simulink model "tqdtqr_rebuild_V3"  (R2021b)
settings: Solver=VariableStepAuto  StartTime=0.0  StopTime=10.0  RelTol=1e-3
undefined symbols (not defined in the file): ATQD_AfterTqMinGain_X_Deg, ATQD_APSCreepBaseTqD_X_kph, ATQD_APSCreepBaseTqD_Y_Deg, ATQD_APSCreepBaseTqR_X_kph, ATQD_APSCreepBaseTqR_Y_Deg, ATQD_APSCreepIterm_X_kph, ATQD_APSCreepIterm_Y_kph, ATQD_APSCreepPterm_X_kph, ATQD_APSCreepPterm_Y_kph, ATQD_APSDecReq_X_kph, ATQD_APSDecReq_Y_mps2, ATQD_APSDecReqCMD_X_kph, ATQD_APSDecReqTs_X_pct, ATQD_APSDecTimeGain_X_Deg, ATQD_APSDecTimeGain_Y_s, ATQD_APSReqLowSpd_X_Deg, ATQD_AutoHoldReleaseBPS_X_Deg, ATQD_AWDLoadTrqnsGain_X_kg, ATQD_AWDLoadTrqnsGain_Y_pct, ATQD_BOSEnBPSPosn_X_kph, ATQD_BOSMap_X_rpm, ATQD_BOSMap_Y_pct, ATQD_CreepBaseTqD_X_kph, ATQD_CreepBaseTqD_Y_Deg, ATQD_CreepBaseTqR_X_kph, ATQD_CreepBaseTqR_Y_Deg, ATQD_CreepBPSDisPosn_X_Deg, ATQD_CreepBPSDisPosnR_X_Deg, ATQD_CreepBPSEnPosn_X_Deg, ATQD_CreepBPSEnPosnR_X_Deg, ATQD_CreepDeltaTq_X_kph, ATQD_CreepIterm_X_kph, ATQD_CreepIterm_Y_kph, ATQD_CreepItermMaxLimit_X_pct, ATQD_CreepPreloadTime_X_kph, ATQD_CreepPreloadTq_X_kph, ATQD_CreepPreloadTq_Y_s, ATQD_CreepProtTq_X_Deg, ATQD_CreepPterm_X_kph, ATQD_CreepPterm_Y_kph, ATQD_CreepRrTqSpRat_X_rpm, ATQD_CreepRrTqSpRat_Y_Nm, ATQD_CreepTargetSpdD_X_pct, ATQD_CreepTargetSpdR_X_pct, ATQD_CreepUpLimitTq_X_rpm, ATQD_DecIneOPDHoldEnDelay_X_Deg, ATQD_DecIneOPDHoldEnDelay_Y_bar, ATQD_ECOTqMapD_X_rpm, ATQD_ECOTqMapD_Y_pct, ATQD_EMTqMapD_X_rpm, ATQD_EMTqMapD_Y_pct, ATQD_EOPDTqMapDCon_X_rpm, ATQD_EOPDTqMapDCon_Y_Deg, ATQD_EstInitVehWeight_X_c, ATQD_FAfterTqCMDGain_X_rpm, ATQD_FAfterTqCMDGain_Y_pct, ATQD_ForceLowSpd_X_Deg, ATQD_ForcePLimitSpd_X_Deg, ATQD_FrLossMAPLowV_X_rpm, ATQD_FrLossMAPLowV_Y_Nm ... (+949)
libraries: simulink x235, hcu_lib x208, tqr x63, tqd x6
(part 26 of 37)

== system tqdtqr_rebuild_V3/Input_Convert/Main function/DriverWhlTqDem function/Driver mode determination/NOLHM ShiftD NRM LV5 ==
  VTQD_ActAPSPosn_pct : Inport
  VTQD_TqTargetShaftSpd_rpm : Inport  Port=2
  VTQD_RL5TqMapDComp_Nm : Inport  Port=3
  Enable : EnablePort
  Add : Sum
  MTQD_NL5TqMapD_Z_Nm1 : Lookup_n-D  BreakpointsForDimension1=ATQD_NL1TqMapD_Y_pct  BreakpointsForDimension2=ATQD_NL1TqMapD_X_rpm  Table=MTQD_NL5TqMapD_Z_Nm  ExtrapMethod=Clip  InternalRulePriority=Speed  RndMeth=Simplest  InputSameDT=on
      settings: InputPortMap=u0,u1
  VTQD_NL5TqMapDOut_Nm : Outport
  wires:
  MTQD_NL5TqMapD_Z_Nm1/1 -> [VTQD_NL5TqMapD_Nm]
  [VTQD_TqTargetShaftSpd_rpm] -> MTQD_NL5TqMapD_Z_Nm1/2
  [VTQD_ActAPSPosn_pct] -> MTQD_NL5TqMapD_Z_Nm1/1
  VTQD_ActAPSPosn_pct/1 -> [VTQD_ActAPSPosn_pct]
  VTQD_TqTargetShaftSpd_rpm/1 -> [VTQD_TqTargetShaftSpd_rpm]
  [VTQD_NL5TqMapD_Nm] -> Add/2
  [VTQD_RL5TqMapDComp_Nm] -> Add/1
  Add/1 -> VTQD_NL5TqMapDOut_Nm/1
  VTQD_RL5TqMapDComp_Nm/1 -> [VTQD_RL5TqMapDComp_Nm]

== system tqdtqr_rebuild_V3/Input_Convert/Main function/DriverWhlTqDem function/Driver mode determination/NOLHM ShiftD NRM OPD ==
  VTQD_ActAPSPosn_pct : Inport
  VTQD_TqTargetShaftSpd_rpm : Inport  Port=2
  VVMC_EstSlope_Deg : Inport  Port=3
  VTQD_APSReqTimer_s : Inport  Port=4
  VTQD_LowIdleAccPedal_flg : Inport  Port=5
  VTQD_OPDHoldEnRel_flg : Inport  Port=6
  VTQD_OPDHoldActRelTq_Nm : Inport  Port=7
  VTQD_VehActSpd_kph : Inport  Port=8
  VTQD_SlopeUp_flg : Inport  Port=9
  Enable : EnablePort
  AND : Logic  AllPortsSameDT=off  OutDataTypeStr=boolean
  Add : Sum
  Constant1 : Constant  Value=ZERO_FLOAT
  Constant2 : Constant  Value=KTQD_OPDHTqDisComSpd_kph
  Constant3 : Constant  Value=KTQD_OPDHTqDisAPSPosn_pct
  Constant9 : Constant  Value=KTQD_APSReqDelayTime_s
  Detect Increase : simulink/Logic and Bit Operations/Detect Increase  vinit=0.0  OutDataTypeStr=boolean
  MTQD_NOPDTqMapDCon_Z_Nm : Lookup_n-D  BreakpointsForDimension1=ATQD_NOPDTqMapDCon_Y_Deg  BreakpointsForDimension2=ATQD_NOPDTqMapDCon_X_rpm  Table=MTQD_NOPDTqMapDCon_Z_Nm  ExtrapMethod=Clip  InternalRulePriority=Speed  RndMeth=Simplest  InputSameDT=on
      settings: InputPortMap=u0,u1
  MTQD_NOPDTqMapD_Z_Nm1 : Lookup_n-D  BreakpointsForDimension1=ATQD_NL1TqMapD_Y_pct  BreakpointsForDimension2=ATQD_NL1TqMapD_X_rpm  Table=MTQD_NOPDTqMapD_Z_Nm  ExtrapMethod=Clip  InternalRulePriority=Speed  RndMeth=Simplest  InputSameDT=on
      settings: InputPortMap=u0,u1
  Max : MinMax  Function=max  Inputs=2
  NOT : Logic  Operator=NOT  AllPortsSameDT=off  OutDataTypeStr=boolean
  OR : Logic  Operator=OR  Inputs=3  AllPortsSameDT=off  OutDataTypeStr=boolean
  OR1 : Logic  Operator=OR  AllPortsSameDT=off  OutDataTypeStr=boolean
  Relational Operator : RelationalOperator  Operator=>  OutDataTypeStr=boolean  RndMeth=Simplest
  Relational Operator1 : RelationalOperator  OutDataTypeStr=boolean  RndMeth=Simplest
  Relational Operator2 : RelationalOperator  OutDataTypeStr=boolean  RndMeth=Simplest
  SR_Latch : hcu_lib/Basic_Blocks/SR_Latch
  Switch : Switch  Criteria=u2 ~= 0
      settings: AttributesFormatString=%<Criteria>
  Switch1 : Switch  Criteria=u2 ~= 0
      settings: AttributesFormatString=%<Criteria>
  VTQD_NOPDTqMapDOut_Nm : Outport
  wires:
  MTQD_NOPDTqMapD_Z_Nm1/1 -> [VTQD_NOPDTqMapD_Nm]
  [VTQD_ActAPSPosn_pct] -> MTQD_NOPDTqMapD_Z_Nm1/1
  [VTQD_TqTargetShaftSpd_rpm] -> MTQD_NOPDTqMapD_Z_Nm1/2
  [VVMC_EstSlope_Deg] -> MTQD_NOPDTqMapDCon_Z_Nm/1
  [VTQD_TqTargetShaftSpd_rpm] -> MTQD_NOPDTqMapDCon_Z_Nm/2
  MTQD_NOPDTqMapDCon_Z_Nm/1 -> [VTQD_NOPDTqMapDCon_Nm]
  VTQD_ActAPSPosn_pct/1 -> [VTQD_ActAPSPosn_pct]
  VTQD_TqTargetShaftSpd_rpm/1 -> [VTQD_TqTargetShaftSpd_rpm]
  VVMC_EstSlope_Deg/1 -> [VVMC_EstSlope_Deg]
  VTQD_APSReqTimer_s/1 -> [VTQD_APSReqTimer_s]
  VTQD_LowIdleAccPedal_flg/1 -> [VTQD_LowIdleAccPedal_flg]
  VTQD_OPDHoldEnRel_flg/1 -> [VTQD_OPDHoldEnRel_flg]
  VTQD_OPDHoldActRelTq_Nm/1 -> [VTQD_OPDHoldActRelTq_Nm]
  VTQD_VehActSpd_kph/1 -> [VTQD_VehActSpd_kph]
  VTQD_SlopeUp_flg/1 -> [VTQD_SlopeUp_flg]
  AND/1 -> OR1/1
  Constant3/1 -> Relational Operator1/2
  [VTQD_ActAPSPosn_pct] -> Relational Operator1/1
  Constant1/1 -> Switch/1
  [VTQD_LowIdleAccPedal_flg] -> OR/1
  OR1/1 -> Switch/2
  NOT/1 -> OR/3
  Max/1 -> Switch1/1
  [VTQD_LowIdleAccPedal_flg] -> AND/2
  Relational Operator/1 -> OR/2
  Constant2/1 -> Relational Operator/2
  Relational Operator2/1 -> AND/1
  [VTQD_NOPDTqMapD_Nm] -> Add/1
  [VTQD_APSReqTimer_s] -> Relational Operator2/1
  OR/1 -> SR_Latch/2
  Relational Operator1/1 -> OR1/2
  Detect Increase/1 -> SR_Latch/1
  Constant9/1 -> Relational Operator2/2
  Add/1 -> Max/1, Switch1/3  "VTQD_NOPDActTqMapD_Nm"
  SR_Latch/1 -> Switch1/2  "VTQD_OPDHoldRelPedTq_flg"
  Switch/1 -> Add/2
  [VTQD_NOPDTqMapDCon_Nm] -> Switch/3
  [VTQD_OPDHoldActRelTq_Nm] -> Max/2
  [VTQD_OPDHoldEnRel_flg] -> Detect Increase/1
  [VTQD_VehActSpd_kph] -> Relational Operator/1
  [VTQD_SlopeUp_flg] -> NOT/1
  Switch1/1 -> VTQD_NOPDTqMapDOut_Nm/1

== system tqdtqr_rebuild_V3/Input_Convert/Main function/DriverWhlTqDem function/Driver mode determination/NOLHM ShiftD Sport Invalid ==
  VTQD_ActAPSPosn_pct : Inport
  VTQD_TqTargetShaftSpd_rpm : Inport  Port=2
  Enable : EnablePort
  MTQD_SL1TqMapD_Z_Nm : Lookup_n-D  BreakpointsForDimension1=ATQD_SL1TqMapD_Y_pct  BreakpointsForDimension2=ATQD_SL1TqMapD_X_rpm  Table=MTQD_SL1TqMapD_Z_Nm  ExtrapMethod=Clip  InternalRulePriority=Speed  RndMeth=Simplest  InputSameDT=on
      settings: InputPortMap=u0,u1
  VTQD_SLTqMapDOutInv_Nm : Outport
  wires:
  MTQD_SL1TqMapD_Z_Nm/1 -> [VTQD_SL1TqMapD_Nm]
  [VTQD_TqTargetShaftSpd_rpm] -> MTQD_SL1TqMapD_Z_Nm/2
  [VTQD_ActAPSPosn_pct] -> MTQD_SL1TqMapD_Z_Nm/1
  VTQD_ActAPSPosn_pct/1 -> [VTQD_ActAPSPosn_pct]
  VTQD_TqTargetShaftSpd_rpm/1 -> [VTQD_TqTargetShaftSpd_rpm]
  [VTQD_SL1TqMapD_Nm] -> VTQD_SLTqMapDOutInv_Nm/1

== system tqdtqr_rebuild_V3/Input_Convert/Main function/DriverWhlTqDem function/Driver mode determination/NOLHM ShiftD Sport LV1 ==
  VTQD_ActAPSPosn_pct : Inport
  VTQD_TqTargetShaftSpd_rpm : Inport  Port=2
  VTQD_RL1TqMapDComp_Nm : Inport  Port=3
  Enable : EnablePort
  Add : Sum
  MTQD_SL1TqMapD_Z_Nm : Lookup_n-D  BreakpointsForDimension1=ATQD_SL1TqMapD_Y_pct  BreakpointsForDimension2=ATQD_SL1TqMapD_X_rpm  Table=MTQD_SL1TqMapD_Z_Nm  ExtrapMethod=Clip  InternalRulePriority=Speed  RndMeth=Simplest  InputSameDT=on
      settings: InputPortMap=u0,u1
  VTQD_SL1TqMapDOut_Nm : Outport
  wires:
  MTQD_SL1TqMapD_Z_Nm/1 -> [VTQD_SL1TqMapD_Nm]
  [VTQD_TqTargetShaftSpd_rpm] -> MTQD_SL1TqMapD_Z_Nm/2
  [VTQD_ActAPSPosn_pct] -> MTQD_SL1TqMapD_Z_Nm/1
  [VTQD_SL1TqMapD_Nm] -> Add/2
  [VTQD_RL1TqMapDComp_Nm] -> Add/1
  Add/1 -> VTQD_SL1TqMapDOut_Nm/1
  VTQD_ActAPSPosn_pct/1 -> [VTQD_ActAPSPosn_pct]
  VTQD_TqTargetShaftSpd_rpm/1 -> [VTQD_TqTargetShaftSpd_rpm]
  VTQD_RL1TqMapDComp_Nm/1 -> [VTQD_RL1TqMapDComp_Nm]

== system tqdtqr_rebuild_V3/Input_Convert/Main function/DriverWhlTqDem function/Driver mode determination/NOLHM ShiftD Sport LV2 ==
  VTQD_ActAPSPosn_pct : Inport
  VTQD_TqTargetShaftSpd_rpm : Inport  Port=2
  VTQD_RL2TqMapDComp_Nm : Inport  Port=3
  Enable : EnablePort
  Add : Sum
  MTQD_SL2TqMapD_Z_Nm : Lookup_n-D  BreakpointsForDimension1=ATQD_SL1TqMapD_Y_pct  BreakpointsForDimension2=ATQD_SL1TqMapD_X_rpm  Table=MTQD_SL2TqMapD_Z_Nm  ExtrapMethod=Clip  InternalRulePriority=Speed  RndMeth=Simplest  InputSameDT=on
      settings: InputPortMap=u0,u1
  VTQD_SL2TqMapDOut_Nm : Outport
  wires:
  [VTQD_ActAPSPosn_pct] -> MTQD_SL2TqMapD_Z_Nm/1
  MTQD_SL2TqMapD_Z_Nm/1 -> [VTQD_SL2TqMapD_Nm]
  [VTQD_TqTargetShaftSpd_rpm] -> MTQD_SL2TqMapD_Z_Nm/2
  VTQD_ActAPSPosn_pct/1 -> [VTQD_ActAPSPosn_pct]
  VTQD_TqTargetShaftSpd_rpm/1 -> [VTQD_TqTargetShaftSpd_rpm]
  [VTQD_RL2TqMapDComp_Nm] -> Add/1
  [VTQD_SL2TqMapD_Nm] -> Add/2
  Add/1 -> VTQD_SL2TqMapDOut_Nm/1
  VTQD_RL2TqMapDComp_Nm/1 -> [VTQD_RL2TqMapDComp_Nm]

== system tqdtqr_rebuild_V3/Input_Convert/Main function/DriverWhlTqDem function/Driver mode determination/NOLHM ShiftD Sport LV3 ==
  VTQD_ActAPSPosn_pct : Inport
  VTQD_TqTargetShaftSpd_rpm : Inport  Port=2
  VTQD_RL3TqMapDComp_Nm : Inport  Port=3
  Enable : EnablePort
  Add : Sum
  MTQD_SL3TqMapD_Z_Nm : Lookup_n-D  BreakpointsForDimension1=ATQD_SL1TqMapD_Y_pct  BreakpointsForDimension2=ATQD_SL1TqMapD_X_rpm  Table=MTQD_SL3TqMapD_Z_Nm  ExtrapMethod=Clip  InternalRulePriority=Speed  RndMeth=Simplest  InputSameDT=on
      settings: InputPortMap=u0,u1
  VTQD_SL3TqMapDOut_Nm : Outport
  wires:
  [VTQD_TqTargetShaftSpd_rpm] -> MTQD_SL3TqMapD_Z_Nm/2
  [VTQD_ActAPSPosn_pct] -> MTQD_SL3TqMapD_Z_Nm/1
  MTQD_SL3TqMapD_Z_Nm/1 -> [VTQD_SL3TqMapD_Nm]
  VTQD_ActAPSPosn_pct/1 -> [VTQD_ActAPSPosn_pct]
  VTQD_TqTargetShaftSpd_rpm/1 -> [VTQD_TqTargetShaftSpd_rpm]
  Add/1 -> VTQD_SL3TqMapDOut_Nm/1
  [VTQD_RL3TqMapDComp_Nm] -> Add/1
  [VTQD_SL3TqMapD_Nm] -> Add/2
  VTQD_RL3TqMapDComp_Nm/1 -> [VTQD_RL3TqMapDComp_Nm]

== system tqdtqr_rebuild_V3/Input_Convert/Main function/DriverWhlTqDem function/Driver mode determination/NOLHM ShiftD Sport LV4 ==
  VTQD_ActAPSPosn_pct : Inport
  VTQD_TqTargetShaftSpd_rpm : Inport  Port=2
  VTQD_RL4TqMapDComp_Nm : Inport  Port=3
  Enable : EnablePort
  Add : Sum
  MTQD_SL4TqMapD_Z_Nm : Lookup_n-D  BreakpointsForDimension1=ATQD_SL1TqMapD_Y_pct  BreakpointsForDimension2=ATQD_SL1TqMapD_X_rpm  Table=MTQD_SL4TqMapD_Z_Nm  ExtrapMethod=Clip  InternalRulePriority=Speed  RndMeth=Simplest  InputSameDT=on
      settings: InputPortMap=u0,u1
  VTQD_SL4TqMapDOut_Nm : Outport
  wires:
  [VTQD_ActAPSPosn_pct] -> MTQD_SL4TqMapD_Z_Nm/1
  MTQD_SL4TqMapD_Z_Nm/1 -> [VTQD_SL4TqMapD_Nm]
  [VTQD_TqTargetShaftSpd_rpm] -> MTQD_SL4TqMapD_Z_Nm/2
  VTQD_ActAPSPosn_pct/1 -> [VTQD_ActAPSPosn_pct]
  VTQD_TqTargetShaftSpd_rpm/1 -> [VTQD_TqTargetShaftSpd_rpm]
  [VTQD_RL4TqMapDComp_Nm] -> Add/1
  [VTQD_SL4TqMapD_Nm] -> Add/2
  Add/1 -> VTQD_SL4TqMapDOut_Nm/1
  VTQD_RL4TqMapDComp_Nm/1 -> [VTQD_RL4TqMapDComp_Nm]

== system tqdtqr_rebuild_V3/Input_Convert/Main function/DriverWhlTqDem function/Driver mode determination/NOLHM ShiftD Sport LV5 ==
  VTQD_ActAPSPosn_pct : Inport
  VTQD_TqTargetShaftSpd_rpm : Inport  Port=2
  VTQD_RL5TqMapDComp_Nm : Inport  Port=3
  Enable : EnablePort
  Add : Sum
  MTQD_SL5TqMapD_Z_Nm : Lookup_n-D  BreakpointsForDimension1=ATQD_SL1TqMapD_Y_pct  BreakpointsForDimension2=ATQD_SL1TqMapD_X_rpm  Table=MTQD_SL5TqMapD_Z_Nm  ExtrapMethod=Clip  InternalRulePriority=Speed  RndMeth=Simplest  InputSameDT=on
      settings: InputPortMap=u0,u1
  VTQD_SL5TqMapDOut_Nm : Outport
  wires:
  MTQD_SL5TqMapD_Z_Nm/1 -> [VTQD_SL5TqMapD_Nm]
  [VTQD_TqTargetShaftSpd_rpm] -> MTQD_SL5TqMapD_Z_Nm/2
  [VTQD_ActAPSPosn_pct] -> MTQD_SL5TqMapD_Z_Nm/1
  VTQD_ActAPSPosn_pct/1 -> [VTQD_ActAPSPosn_pct]
  VTQD_TqTargetShaftSpd_rpm/1 -> [VTQD_TqTargetShaftSpd_rpm]
  [VTQD_RL5TqMapDComp_Nm] -> Add/1
  [VTQD_SL5TqMapD_Nm] -> Add/2
  Add/1 -> VTQD_SL5TqMapDOut_Nm/1
  VTQD_RL5TqMapDComp_Nm/1 -> [VTQD_RL5TqMapDComp_Nm]

== system tqdtqr_rebuild_V3/Input_Convert/Main function/DriverWhlTqDem function/Driver mode determination/NOLHM ShiftD Sport OPD ==
  VTQD_ActAPSPosn_pct : Inport
  VTQD_TqTargetShaftSpd_rpm : Inport  Port=2
  VVMC_EstSlope_Deg : Inport  Port=3
  VTQD_APSReqTimer_s : Inport  Port=4
  VTQD_LowIdleAccPedal_flg : Inport  Port=5
  VTQD_OPDHoldEnRel_flg : Inport  Port=6
  VTQD_OPDHoldActRelTq_Nm : Inport  Port=7
  VTQD_VehActSpd_kph : Inport  Port=8
  VTQD_SlopeUp_flg : Inport  Port=9
  Enable : EnablePort
  AND : Logic  AllPortsSameDT=off  OutDataTypeStr=boolean
  Add : Sum
  Constant1 : Constant  Value=ZERO_FLOAT
  Constant2 : Constant  Value=KTQD_OPDHTqDisComSpd_kph
  Constant4 : Constant  Value=KTQD_OPDHTqDisAPSPosn_pct
  Constant9 : Constant  Value=KTQD_APSReqDelayTime_s
  Detect Increase : simulink/Logic and Bit Operations/Detect Increase  vinit=0.0  OutDataTypeStr=boolean
  MTQD_SOPDTqMapDCon_Z_Nm : Lookup_n-D  BreakpointsForDimension1=ATQD_SOPDTqMapDCon_Y_Deg  BreakpointsForDimension2=ATQD_SOPDTqMapDCon_X_rpm  Table=MTQD_SOPDTqMapDCon_Z_Nm  ExtrapMethod=Clip  InternalRulePriority=Speed  RndMeth=Simplest  InputSameDT=on
      settings: InputPortMap=u0,u1
  MTQD_SOPDTqMapD_Z_Nm : Lookup_n-D  BreakpointsForDimension1=ATQD_SL1TqMapD_Y_pct  BreakpointsForDimension2=ATQD_SL1TqMapD_X_rpm  Table=MTQD_SOPDTqMapD_Z_Nm  ExtrapMethod=Clip  InternalRulePriority=Speed  RndMeth=Simplest  InputSameDT=on
      settings: InputPortMap=u0,u1
  Max : MinMax  Function=max  Inputs=2
  NOT : Logic  Operator=NOT  AllPortsSameDT=off  OutDataTypeStr=boolean
  OR : Logic  Operator=OR  Inputs=3  AllPortsSameDT=off  OutDataTypeStr=boolean
  OR1 : Logic  Operator=OR  AllPortsSameDT=off  OutDataTypeStr=boolean
  Relational Operator : RelationalOperator  Operator=>  OutDataTypeStr=boolean  RndMeth=Simplest
  Relational Operator2 : RelationalOperator  OutDataTypeStr=boolean  RndMeth=Simplest
  Relational Operator3 : RelationalOperator  OutDataTypeStr=boolean  RndMeth=Simplest
  SR_Latch : hcu_lib/Basic_Blocks/SR_Latch
  Switch : Switch  Criteria=u2 ~= 0
      settings: AttributesFormatString=%<Criteria>
  Switch1 : Switch  Criteria=u2 ~= 0
      settings: AttributesFormatString=%<Criteria>
  VTQD_SOPDTqMapDOut_Nm : Outport
  wires:
  MTQD_SOPDTqMapD_Z_Nm/1 -> [VTQD_SOPDTqMapD_Nm]
  [VVMC_EstSlope_Deg] -> MTQD_SOPDTqMapDCon_Z_Nm/1
  [VTQD_TqTargetShaftSpd_rpm] -> MTQD_SOPDTqMapDCon_Z_Nm/2
  MTQD_SOPDTqMapDCon_Z_Nm/1 -> [VTQD_SOPDTqMapDCon_Nm]
  [VTQD_ActAPSPosn_pct] -> MTQD_SOPDTqMapD_Z_Nm/1
  [VTQD_TqTargetShaftSpd_rpm] -> MTQD_SOPDTqMapD_Z_Nm/2
  VTQD_ActAPSPosn_pct/1 -> [VTQD_ActAPSPosn_pct]
  VTQD_TqTargetShaftSpd_rpm/1 -> [VTQD_TqTargetShaftSpd_rpm]
  VVMC_EstSlope_Deg/1 -> [VVMC_EstSlope_Deg]
  [VTQD_ActAPSPosn_pct] -> Relational Operator3/1
  [VTQD_SOPDTqMapDCon_Nm] -> Switch/3
  OR1/1 -> Switch/2
  AND/1 -> OR1/1
  Relational Operator3/1 -> OR1/2
  Constant4/1 -> Relational Operator3/2
  [VTQD_SOPDTqMapD_Nm] -> Add/1
  [VTQD_APSReqTimer_s] -> Relational Operator2/1
  Constant9/1 -> Relational Operator2/2
  Relational Operator2/1 -> AND/1
  [VTQD_LowIdleAccPedal_flg] -> AND/2
  Switch/1 -> Add/2
  Constant1/1 -> Switch/1
  VTQD_APSReqTimer_s/1 -> [VTQD_APSReqTimer_s]
  VTQD_LowIdleAccPedal_flg/1 -> [VTQD_LowIdleAccPedal_flg]
  VTQD_OPDHoldEnRel_flg/1 -> [VTQD_OPDHoldEnRel_flg]
  VTQD_OPDHoldActRelTq_Nm/1 -> [VTQD_OPDHoldActRelTq_Nm]
  VTQD_VehActSpd_kph/1 -> [VTQD_VehActSpd_kph]
  VTQD_SlopeUp_flg/1 -> [VTQD_SlopeUp_flg]
  [VTQD_SlopeUp_flg] -> NOT/1
  SR_Latch/1 -> Switch1/2
  Constant2/1 -> Relational Operator/2
  [VTQD_OPDHoldEnRel_flg] -> Detect Increase/1
  Add/1 -> Switch1/3, Max/1  "VTQD_SOPDActTqMapD_Nm"
  [VTQD_LowIdleAccPedal_flg] -> OR/1
  OR/1 -> SR_Latch/2
  Relational Operator/1 -> OR/2
  NOT/1 -> OR/3
  [VTQD_VehActSpd_kph] -> Relational Operator/1
  Max/1 -> Switch1/1
  Switch1/1 -> VTQD_SOPDTqMapDOut_Nm/1
  [VTQD_OPDHoldActRelTq_Nm] -> Max/2
  Detect Increase/1 -> SR_Latch/1

== system tqdtqr_rebuild_V3/Input_Convert/Main function/DriverWhlTqDem function/Driver mode determination/NoLHM ShiftD Rock ==
  VTQD_TqTargetShaftSpd_rpm : Inport
  VTQD_ActAPSPosn_pct : Inport  Port=2
  Enable : EnablePort
  MTQD_EMTqMapD_Z_Nm : Lookup_n-D  BreakpointsForDimension1=ATQD_EMTqMapD_Y_pct  BreakpointsForDimension2=ATQD_EMTqMapD_X_rpm  Table=MTQD_EMTqMapD_Z_Nm  ExtrapMethod=Clip  InternalRulePriority=Speed  RndMeth=Simplest  InputSameDT=on
      settings: InputPortMap=u0,u1
  VTQD_WhlTqRockMode_Nm : Outport
  wires:
  VTQD_ActAPSPosn_pct/1 -> [VTQD_ActAPSPosn_pct]
  VTQD_TqTargetShaftSpd_rpm/1 -> [VTQD_TqTargetShaftSpd_rpm]
  MTQD_EMTqMapD_Z_Nm/1 -> VTQD_WhlTqRockMode_Nm/1
  [VTQD_TqTargetShaftSpd_rpm] -> MTQD_EMTqMapD_Z_Nm/2
  [VTQD_ActAPSPosn_pct] -> MTQD_EMTqMapD_Z_Nm/1

== system tqdtqr_rebuild_V3/Input_Convert/Main function/DriverWhlTqDem function/Driver mode determination/NoLHM ShiftD Snow ==
  VTQD_TqTargetShaftSpd_rpm : Inport
  VTQD_ActAPSPosn_pct : Inport  Port=2
  VTQD_RegenMode_enum : Inport  Port=3
  VTQD_PreDecTqLowLim_Nm : Inport  Port=4
  Enable : EnablePort
  Constant1 : Constant  Value=ZERO_FLOAT
  Constant2 : Constant  Value=ENUM_REGENLEVEL_LV1
  Constant3 : Constant  Value=KTQD_PedalMapRDCUpLim_Nm
  Equal : RelationalOperator  Operator===  OutDataTypeStr=boolean  RndMeth=Simplest
  MTQD_SN1TqMapD_Z_Nm : Lookup_n-D  BreakpointsForDimension1=ATQD_SNTqMapD_Y_pct  BreakpointsForDimension2=ATQD_SNTqMapD_X_rpm  Table=MTQD_SNTqMapD_Z_Nm  ExtrapMethod=Clip  InternalRulePriority=Speed  RndMeth=Simplest  InputSameDT=on
      settings: InputPortMap=u0,u1
  Saturation Dynamic : simulink/Discontinuities/Saturation Dynamic  OutMin=[]  OutMax=[]  OutDataTypeStr=Inherit: Same as second input  OutDataType=fixdt(1, 16)  OutScaling=2^-10  DoSatur=off
  Switch : Switch  Criteria=u2 ~= 0
      settings: AttributesFormatString=%<Criteria>
  VTQD_WhlTqSnowMode_Nm : Outport
  wires:
  VTQD_PreDecTqLowLim_Nm/1 -> [VTQD_PreDecTqLowLim_Nm]
  VTQD_ActAPSPosn_pct/1 -> [VTQD_ActAPSPosn_pct]
  VTQD_RegenMode_enum/1 -> [VTQD_RegenMode_enum]
  VTQD_TqTargetShaftSpd_rpm/1 -> [VTQD_TqTargetShaftSpd_rpm]
  [VTQD_PreDecTqLowLim_Nm] -> Switch/3
  Saturation Dynamic/1 -> VTQD_WhlTqSnowMode_Nm/1
  [VTQD_RegenMode_enum] -> Equal/1
  [VTQD_SNTqMapD_Nm] -> Saturation Dynamic/2
  [VTQD_TqTargetShaftSpd_rpm] -> MTQD_SN1TqMapD_Z_Nm/2
  Switch/1 -> Saturation Dynamic/3
  Equal/1 -> Switch/2
  Constant2/1 -> Equal/2
  MTQD_SN1TqMapD_Z_Nm/1 -> [VTQD_SNTqMapD_Nm]  "VTQD_SNTqMapD_Nm"
  Constant3/1 -> Saturation Dynamic/1
  [VTQD_ActAPSPosn_pct] -> MTQD_SN1TqMapD_Z_Nm/1
  Constant1/1 -> Switch/1

== system tqdtqr_rebuild_V3/Input_Convert/Main function/DriverWhlTqDem function/Driver mode determination/NoLHM ShiftProN ==
  Enable : EnablePort
  Constant : Constant  Value=ZERO_FLOAT
  VTQD_PedalMapWhlTqPorN_Nm : Outport
  wires:
  Constant/1 -> VTQD_PedalMapWhlTqPorN_Nm/1

== system tqdtqr_rebuild_V3/Input_Convert/Main function/DriverWhlTqDem function/Driver mode determination/NoLHM ShiftR ==
  VTQD_ActAPSPosn_pct : Inport
  VTQD_TqTargetShaftSpd_rpm : Inport  Port=2
  VTQD_DOALatchReq_flg : Inport  Port=3
  Enable : EnablePort
  AND : Logic  AllPortsSameDT=off  OutDataTypeStr=boolean
  Constant : Constant  Value=KTQD_DOAOPDReqSW_flg
  If : If  IfExpression="u1 ~=  0"
  If Action Subsystem : Subsystem  AncestorBlock=tqd_newcode/TQD/TorqueDemand/TorqueModule/DriverWhlTqDem/PedalMapWhlTq/NoLHM/ShiftR/If Action Subsystem  TreatAsAtomicUnit=on
  If Action Subsystem1 : Subsystem  AncestorBlock=tqd_newcode/TQD/TorqueDemand/TorqueModule/DriverWhlTqDem/PedalMapWhlTq/NoLHM/ShiftR/If Action Subsystem1  TreatAsAtomicUnit=on
  Merge : Merge
  VTQD_PedalMapWhlTqR_Nm : Outport
  wires:
  VTQD_TqTargetShaftSpd_rpm/1 -> [VTQD_TqTargetShaftSpd_rpm]
  VTQD_ActAPSPosn_pct/1 -> [VTQD_ActAPSPosn_pct]
  [VTQD_NRMTqMapR_Nm] -> VTQD_PedalMapWhlTqR_Nm/1
  If/2 -> If Action Subsystem1/Action
  If Action Subsystem1/1(Out1) -> Merge/2
  [VTQD_DOALatchReq_flg] -> AND/1
  AND/1 -> If/1
  Constant/1 -> AND/2
  [VTQD_ActAPSPosn_pct] -> If Action Subsystem/1(In1)
  [VTQD_ActAPSPosn_pct] -> If Action Subsystem1/1(In1)
  If/1 -> If Action Subsystem/Action
  Merge/1 -> [VTQD_NRMTqMapR_Nm]
  [VTQD_TqTargetShaftSpd_rpm] -> If Action Subsystem/2(Inport)
  If Action Subsystem/1(Out1) -> Merge/1
  [VTQD_TqTargetShaftSpd_rpm] -> If Action Subsystem1/2(Inport)
  VTQD_DOALatchReq_flg/1 -> [VTQD_DOALatchReq_flg]

== system tqdtqr_rebuild_V3/Input_Convert/Main function/DriverWhlTqDem function/Pedal G-Control Mode/Active Determination ==
  VINP_SCPSystemMode_enum : Inport
  VPMM_PwrSta_enum : Inport  Port=2
  VTQD_GearActualPosn_enum : Inport  Port=3
  VTQD_RegenMode_enum : Inport  Port=4
  VINP_SWC2RCustomizeSta_flg : Inport  Port=5
  task_time_s : Inport  Port=6
  VINP_SWCResUpSta_flg : Inport  Port=7
  AND : Logic  Inputs=4  AllPortsSameDT=off  OutDataTypeStr=boolean
  AND1 : Logic  AllPortsSameDT=off  OutDataTypeStr=boolean
  AND2 : Logic  AllPortsSameDT=off  OutDataTypeStr=boolean
  AND3 : Logic  AllPortsSameDT=off  OutDataTypeStr=boolean
  AND4 : Logic  Inputs=3  AllPortsSameDT=off  OutDataTypeStr=boolean
  Constant1 : Constant  Value=ENUM_SYSMODE_ENGINEERING
  Constant10 : Constant  Value=ENUM_GEARACTUALPOSN_R
  Constant11 : Constant  Value=KTQD_PedAccTqEn_flg_ovrdflg
  Constant12 : Constant  Value=KTQD_PedGControlModeSW_flg
  Constant13 : Constant  Value=KTQD_PedAccTqEn_flg_ovrdval
  Constant2 : Constant  Value=ENUM_POWERSTA_READY
  Constant21 : Constant  Value=ENUM_SYSMODE_DEVELOPING
  Constant3 : Constant  Value=ENUM_GEARACTUALPOSN_R
  Constant4 : Constant  Value=ENUM_REGENLEVEL_OPD
  Constant5 : Constant  Value=KTQD_PedGControlModeSW_flg
  Constant6 : Constant  Value=KTQD_PedGControlTrigTime_s
  Constant7 : Constant  Value=ENUM_SYSMODE_ENGINEERING
  Constant8 : Constant  Value=ENUM_POWERSTA_READY
  Constant9 : Constant  Value=ENUM_SYSMODE_DEVELOPING
  Delay : Delay  DelayLength=1  InitialCondition=boolean(0)
      settings: AttributesFormatString=%<InitialCondition>
  DelayEnable3 : hcu_lib/Basic_Blocks/DelayEnable
  Detect Decrease : simulink/Logic and Bit Operations/Detect Decrease  vinit=0.0  OutDataTypeStr=boolean
  Detect Decrease5 : simulink/Logic and Bit Operations/Detect Decrease  vinit=0.0  OutDataTypeStr=boolean
  Equal{,1..2,4..7} (7 alike) : RelationalOperator  Operator===  OutDataTypeStr=boolean  RndMeth=Simplest
  Equal3 : RelationalOperator  Operator=~=  OutDataTypeStr=boolean  RndMeth=Simplest
  Equal8 : RelationalOperator  Operator=~=  OutDataTypeStr=boolean  RndMeth=Simplest
  OR : Logic  Operator=OR  Inputs=3  AllPortsSameDT=off  OutDataTypeStr=boolean
  OR1 : Logic  Operator=OR  Inputs=3  AllPortsSameDT=off  OutDataTypeStr=boolean
  OR2 : Logic  Operator=OR  AllPortsSameDT=off  OutDataTypeStr=boolean
  OR3 : Logic  Operator=OR  AllPortsSameDT=off  OutDataTypeStr=boolean
  SR_Latch3 : hcu_lib/Basic_Blocks/SR_Latch
  Switch : Switch  Criteria=u2 ~= 0
      settings: AttributesFormatString=%<Criteria>
  VTQD_PedAccTqEn_flg : Outport
  wires:
  Constant2/1 -> Equal2/2
  Constant5/1 -> OR/3
  Constant21/1 -> Equal/2
  Constant1/1 -> Equal1/2
  Equal2/1 -> AND/2
  [VINP_SCPSystemMode_enum] -> Equal1/1
  Equal1/1 -> OR/2
  [VTQD_GearActualPosn_enum] -> Equal3/1
  Equal4/1 -> AND/4
  Constant3/1 -> Equal3/2
  Equal3/1 -> AND/3
  [VPMM_PwrSta_enum] -> Equal2/1
  Equal/1 -> OR/1
  Constant4/1 -> Equal4/2
  OR/1 -> AND/1
  [VTQD_RegenMode_enum] -> Equal4/1
  AND/1 -> [VTQD_PedGControlAllow_flg]  "VTQD_PedGControlAllow_flg"
  [VINP_SCPSystemMode_enum] -> Equal/1
  Detect Decrease5/1 -> AND1/1, SR_Latch3/1
  Delay/1 -> AND1/2
  Constant6/1 -> DelayEnable3/2
  [task_time_s] -> DelayEnable3/3
  DelayEnable3/1 -> Detect Decrease5/1  "VTQD_PedGControlTrig_flg"
  SR_Latch3/1 -> AND2/1
  [VTQD_PedAccTqOperate_flg] -> AND2/2
  [VTQD_PedAccTqEn_flg] -> Delay/1
  VINP_SCPSystemMode_enum/1 -> [VINP_SCPSystemMode_enum]
  VPMM_PwrSta_enum/1 -> [VPMM_PwrSta_enum]
  VTQD_GearActualPosn_enum/1 -> [VTQD_GearActualPosn_enum]
  VTQD_RegenMode_enum/1 -> [VTQD_RegenMode_enum]
  VINP_SWC2RCustomizeSta_flg/1 -> [VINP_SWC2RCustomizeSta_flg]
  task_time_s/1 -> [task_time_s]
  [VTQD_PedAccTqEn_flg] -> VTQD_PedAccTqEn_flg/1
  [VTQD_PedGControlAllow_flg] -> AND3/1
  AND3/1 -> DelayEnable3/1
  [VINP_SCPSystemMode_enum] -> Equal5/1
  OR1/1 -> [VTQD_PedGControlModeSW_flg], AND4/1  "VTQD_PedGControlModeSW_flg"
  Equal5/1 -> OR1/1
  [VPMM_PwrSta_enum] -> Equal7/1
  Equal8/1 -> AND4/3
  Constant10/1 -> Equal8/2
  [VTQD_GearActualPosn_enum] -> Equal8/1
  Equal6/1 -> OR1/2
  [VINP_SCPSystemMode_enum] -> Equal6/1
  Equal7/1 -> AND4/2
  Constant7/1 -> Equal6/2
  Constant9/1 -> Equal5/2
  Constant12/1 -> OR1/3
  Constant8/1 -> Equal7/2
  AND4/1 -> [VTQD_PedAccTqOperate_flg]  "VTQD_PedAccTqOperate_flg"
  AND1/1 -> OR2/1
  OR2/1 -> SR_Latch3/2
  Detect Decrease/1 -> OR2/2
  [VTQD_PedGControlModeSW_flg] -> Detect Decrease/1
  AND2/1 -> Switch/3
  Switch/1 -> [VTQD_PedAccTqEn_flg]  "VTQD_PedAccTqEn_flg"
  Constant11/1 -> Switch/2
  Constant13/1 -> Switch/1
  VINP_SWCResUpSta_flg/1 -> [VINP_SWCResUpSta_flg]
  OR3/1 -> AND3/2
  [VINP_SWC2RCustomizeSta_flg] -> OR3/1
  [VINP_SWCResUpSta_flg] -> OR3/2

== system tqdtqr_rebuild_V3/Input_Convert/Main function/DriverWhlTqDem function/Pedal G-Control Mode/Torque Calculation ==
  VTQD_ActAPSPosn_pct : Inport
  VTQD_TqTargetShaftSpd_rpm : Inport  Port=2
  VVMC_LongAcc_Gps : Inport  Port=3
  VINP_VehSpeed_kph : Inport  Port=4
  VTQD_PedAccTqEn_flg : Inport  Port=5
  VTQD_GearActualPosn_enum : Inport  Port=6
  VTQD_CreepPrLoadEnable_flg : Inport  Port=7
  VINP_BrkPedalPos_pct : Inport  Port=8
  VINP_IVIPedalGRegenLim_pct : Inport  Port=9
  VVMC_SmartRegenReq_mps2 : Inport  Port=10
  VINP_IVISmartRegenSW_flg : Inport  Port=11
  VINP_IVICreepOnSW_flg : Inport  Port=12
  VTQD_APSReqTimer_s : Inport  Port=13
  AND{,1..3} (4 alike) : Logic  AllPortsSameDT=off  OutDataTypeStr=boolean
  Add : Sum
  Add1 : Sum  Inputs=+-
  Constant1 : Constant  Value=KTQD_PedAccCMDUpLim_mps2
  Constant10 : Constant  Value=KVMC_GravityValue_mps2
  Constant11 : Constant  Value=KTQD_PedAccDevLowLim_mps2
  Constant12 : Constant  Value=ONE_PERCENT
  Constant13 : Constant  Value=KTQD_PedAccBrkEnPos_pct
  Constant14 : Constant  Value=KTQD_PedAccBrkDeltaTq_Nm
  Constant{6..7,15,21} (4 alike) : Constant  Value=ZERO_INT
  Constant16 : Constant  Value=ZERO_FLOAT
  Constant17 : Constant  Value=KTQD_PedAccARgnEnSpd_kph
  Constant18 : Constant  Value=KTQD_PedAccBrkEnPos_pct
  Constant19 : Constant  Value=KTQD_PedAccDevUpLim_mps2
  Constant2 : Constant  Value=KTQD_PedAccCMDLowLim_mps2
  Constant20 : Constant  Value=KTQD_PedAccARgnEnSpd_kph
  Constant22 : Constant  Value=KTQD_APSReqDelayTime_s
  Constant23 : Constant  Value=KTQD_PedAccCMDLowLim_mps2
  Constant3 : Constant  Value=KTQD_PedAccTqUpLim_Nm
  Constant4 : Constant  Value=KTQD_PedAccTqLowLim_Nm
  Constant5 : Constant  Value=KTQD_PedGControlEnSpd_kph
  Constant8 : Constant  Value=ENUM_GEARACTUALPOSN_D
  Constant9 : Constant  Value=ZERO_FLOAT
  Delay : Delay  DelayLength=1
  Delay1 : Delay  DelayLength=1
  Equal : RelationalOperator  Operator===  OutDataTypeStr=boolean  RndMeth=Simplest
  Equal1 : RelationalOperator  OutDataTypeStr=boolean  RndMeth=Simplest
  MTQD_PedAccBrkTq_Y_Nm : Lookup_n-D  NumberOfTableDimensions=1  BreakpointsForDimension1=ATQD_PedAccBrkTq_X_pct  Table=MTQD_PedAccBrkTq_Y_Nm  InternalRulePriority=Speed  RndMeth=Simplest  InputSameDT=on
  MTQD_PedalAccelCMDWC_Z_mps2 : Lookup_n-D  BreakpointsForDimension1=ATQD_PedalAccelCMD_Y_pct  BreakpointsForDimension2=ATQD_PedalAccelCMD_X_rpm  BreakpointsForDimension3=[5, 7]  Table=MTQD_PedalAccelCMDWC_Z_mps2  ExtrapMethod=Clip  InternalRulePriority=Speed  RndMeth=Simplest  InputSameDT=on
      settings: InputPortMap=u0,u1
  MTQD_PedalAccelCMD_Z_mps2 : Lookup_n-D  BreakpointsForDimension1=ATQD_PedalAccelCMD_Y_pct  BreakpointsForDimension2=ATQD_PedalAccelCMD_X_rpm  BreakpointsForDimension3=[5, 7]  Table=MTQD_PedalAccelCMD_Z_mps2  ExtrapMethod=Clip  InternalRulePriority=Speed  RndMeth=Simplest  InputSameDT=on
      settings: InputPortMap=u0,u1
  MTQD_PedalGDeltaTqIGain_Z_Nm : Lookup_n-D  BreakpointsForDimension1=ATQD_PedalGDeltaTqIGain_Y_mps2  BreakpointsForDimension2=ATQD_PedalGDeltaTqIGain_X_kph  Table=MTQD_PedalGDeltaTqIGain_Z_Nm  InternalRulePriority=Speed  RndMeth=Simplest  InputSameDT=on
      settings: InputPortMap=u0,u1
  Max : MinMax  Function=max  Inputs=2
  OR : Logic  Operator=OR  AllPortsSameDT=off  OutDataTypeStr=boolean
  OR1 : Logic  Operator=OR  AllPortsSameDT=off  OutDataTypeStr=boolean
  Product : Product
  Product1 : Product  Inputs=3
  Relational Operator : RelationalOperator  Operator=<=  OutDataTypeStr=boolean  RndMeth=Simplest
  Relational Operator1 : RelationalOperator  Operator=<=  OutDataTypeStr=boolean  RndMeth=Simplest
  Relational Operator3 : RelationalOperator  OutDataTypeStr=boolean  RndMeth=Simplest
  Relational Operator4 : RelationalOperator  OutDataTypeStr=boolean  RndMeth=Simplest
  Relational Operator5 : RelationalOperator  Operator=>  OutDataTypeStr=boolean  RndMeth=Simplest
  Relational Operator6 : RelationalOperator  OutDataTypeStr=boolean  RndMeth=Simplest
  Relational Operator7 : RelationalOperator  Operator=<=  OutDataTypeStr=boolean  RndMeth=Simplest
  Saturation Dynamic{,1..3} (4 alike) : simulink/Discontinuities/Saturation Dynamic  OutMin=[]  OutMax=[]  OutDataTypeStr=Inherit: Same as second input  OutDataType=fixdt(1, 16)  OutScaling=2^-10  DoSatur=off
  Switch{,1..4,6} (6 alike) : Switch  Criteria=u2 ~= 0
      settings: AttributesFormatString=%<Criteria>
  Switch5 : Switch  Criteria=u2 > Threshold
  VTQD_PedalTqCal_Nm : Outport
  wires:
  Saturation Dynamic1/1 -> MTQD_PedalGDeltaTqIGain_Z_Nm/1  "VTQD_PedalAccDev_mps2"
  [VTQD_PedalAccDeltaTq_Nm] -> Add/1
  Constant11/1 -> Saturation Dynamic1/3
  [VTQD_PedalReqAccel_mps2] -> Add1/1
  [VTQD_ActAPSPosn_pct] -> MTQD_PedalAccelCMD_Z_mps2/1
  [VTQD_TqTargetShaftSpd_rpm] -> MTQD_PedalAccelCMD_Z_mps2/2
  Constant6/1 -> Switch/3
  [VVMC_LongAcc_Gps] -> Product/1
  [VINP_VehSpeed_kph] -> MTQD_PedalGDeltaTqIGain_Z_Nm/2
  Add1/1 -> Saturation Dynamic1/2
  Constant19/1 -> Saturation Dynamic1/1
  Constant10/1 -> Product/2
  Constant1/1 -> Saturation Dynamic2/1
  Delay/1 -> [VTQD_LastPedalTqCal_Nm]  "VTQD_LastPedalTqCal_Nm"
  Product/1 -> Add1/2
  Switch/1 -> Saturation Dynamic/2
  Saturation Dynamic2/1 -> [VTQD_PedalReqAccel_mps2]  "VTQD_PedalReqAccel_mps2"
  [VTQD_LastPedalTqCal_Nm] -> Add/2
  VTQD_ActAPSPosn_pct/1 -> [VTQD_ActAPSPosn_pct]
  VTQD_TqTargetShaftSpd_rpm/1 -> [VTQD_TqTargetShaftSpd_rpm]
  VVMC_LongAcc_Gps/1 -> [VVMC_LongAcc_Gps]
  VINP_VehSpeed_kph/1 -> [VINP_VehSpeed_kph]
  VTQD_PedAccTqEn_flg/1 -> [VTQD_PedAccTqEn_flg]
  [VTQD_PedalTqCal_Nm] -> VTQD_PedalTqCal_Nm/1
  [VINP_VehSpeed_kph] -> Relational Operator/1
  Constant5/1 -> Relational Operator/2
  Relational Operator/1 -> AND/1
  Constant4/1 -> Switch1/3
  Constant7/1 -> Switch1/1
  Switch1/1 -> [VTQD_PedAccTqLowLim_Nm]  "VTQD_PedAccTqLowLim_Nm"
  [VTQD_PedAccTqLowLim_Nm] -> Saturation Dynamic/3
  [VTQD_PedAccTqEn_flg] -> AND1/1
  Equal/1 -> AND1/2
  [VTQD_GearActualPosn_enum] -> Equal/1
  Constant8/1 -> Equal/2
  VTQD_GearActualPosn_enum/1 -> [VTQD_GearActualPosn_enum]
  VTQD_CreepPrLoadEnable_flg/1 -> [VTQD_CreepPrLoadEnable_flg]
  Add/1 -> Switch/1
  [VTQD_PedalReqAccel_mps2] -> Relational Operator1/1
  Relational Operator1/1 -> AND/2
  Constant9/1 -> Relational Operator1/2
  AND/1 -> OR1/1
  OR1/1 -> Switch1/2
  Delay1/1 -> OR1/2
  [VTQD_CreepPrLoadEnable_flg] -> Delay1/1
  VINP_BrkPedalPos_pct/1 -> [VINP_BrkPedalPos_pct]
  [VINP_BrkPedalPos_pct] -> Relational Operator3/1
  Constant13/1 -> Relational Operator3/2
  Switch3/1 -> Switch2/1
  Constant14/1 -> Switch3/1
  [VTQD_LastPedalTqCal_Nm] -> Relational Operator4/1
  Relational Operator4/1 -> Switch3/2
  Constant16/1 -> Switch3/3
  Saturation Dynamic/1 -> [VTQD_PedalTqCal_Nm], Delay/1  "VTQD_PedalTqCal_Nm"
  MTQD_PedalGDeltaTqIGain_Z_Nm/1 -> Switch2/3
  Switch2/1 -> [VTQD_PedalAccDeltaTq_Nm]  "VTQD_PedalAccDeltaTq_Nm"
  AND2/1 -> Switch2/2
  Relational Operator3/1 -> AND2/1
  [VINP_VehSpeed_kph] -> Relational Operator5/1
  Constant17/1 -> Relational Operator5/2
  Relational Operator5/1 -> AND2/2
  Relational Operator7/1 -> AND3/2
  Constant20/1 -> Relational Operator7/2
  [VINP_BrkPedalPos_pct] -> Relational Operator6/1
  Constant18/1 -> Relational Operator6/2
  [VINP_VehSpeed_kph] -> Relational Operator7/1
  Relational Operator6/1 -> AND3/1
  AND3/1 -> Switch4/2
  Constant3/1 -> Switch4/3
  Constant21/1 -> Switch4/1
  Switch4/1 -> [VTQD_PedAccTqUpLim_Nm]  "VTQD_PedAccTqUpLim_Nm"
  [VTQD_PedAccTqUpLim_Nm] -> Saturation Dynamic/1
  [VTQD_PedAccBrkTq_Nm] -> Relational Operator4/2
  MTQD_PedAccBrkTq_Y_Nm/1 -> Saturation Dynamic3/2
  Saturation Dynamic3/1 -> [VTQD_PedAccBrkTq_Nm]  "VTQD_PedAccBrkTq_Nm"
  Constant15/1 -> Saturation Dynamic3/1
  [VTQD_PedAccTqLowLim_Nm] -> Saturation Dynamic3/3
  VINP_IVIPedalGRegenLim_pct/1 -> [VINP_IVIPedalGRegenLim_pct]
  [VINP_IVIPedalGRegenLim_pct] -> MTQD_PedAccBrkTq_Y_Nm/1
  Constant2/1 -> Product1/1
  [VINP_IVIPedalGRegenLim_pct] -> Product1/2
  Constant12/1 -> Product1/3
  Product1/1 -> Max/1
  Max/1 -> Saturation Dynamic2/3
  Switch5/1 -> Max/2
  [VVMC_SmartRegenReq_mps2] -> Switch5/1
  Constant23/1 -> Switch5/3
  [VINP_IVISmartRegenSW_flg] -> Switch5/2
  VVMC_SmartRegenReq_mps2/1 -> [VVMC_SmartRegenReq_mps2]
  VINP_IVISmartRegenSW_flg/1 -> [VINP_IVISmartRegenSW_flg]
  MTQD_PedalAccelCMD_Z_mps2/1 -> [VTQD_PedalAccelCMD_mps2]  "VTQD_PedalAccelCMD_mps2"
  MTQD_PedalAccelCMDWC_Z_mps2/1 -> [VTQD_PedalAccelCMDWC_mps2]  "VTQD_PedalAccelCMDWC_mps2"
  [VTQD_TqTargetShaftSpd_rpm] -> MTQD_PedalAccelCMDWC_Z_mps2/2
  [VTQD_ActAPSPosn_pct] -> MTQD_PedalAccelCMDWC_Z_mps2/1
  VINP_IVICreepOnSW_flg/1 -> [VINP_IVICreepOnSW_flg]
  Switch6/1 -> Saturation Dynamic2/2
  [VINP_IVICreepOnSW_flg] -> Switch6/2
  [VTQD_PedalAccelCMD_mps2] -> Switch6/3
  [VTQD_PedalAccelCMDWC_mps2] -> Switch6/1
  VTQD_APSReqTimer_s/1 -> [VTQD_APSReqTimer_s]
  OR/1 -> Switch/2
  AND1/1 -> OR/1
  Equal1/1 -> OR/2
  [VTQD_APSReqTimer_s] -> Equal1/1
  Constant22/1 -> Equal1/2

== system tqdtqr_rebuild_V3/Input_Convert/Main function/DriverWhlTqDem function/PedalMapWhlTq/Triggered Subsystem ==
  in1 : Inport
  In2 : Inport  Port=2
  Trigger : TriggerPort  VariantControl=(inherit)
  Out1 : Outport
  Out2 : Outport  Port=2
  wires:
  in1/1 -> Out1/1
  In2/1 -> Out2/1

== system tqdtqr_rebuild_V3/Input_Convert/Main function/DriverWhlTqDem function/Preload system/New Preload Torque ==
  VTQD_PreLoadHold_flg : Inport
  VTQD_PreLoadHoldtime_s : Inport  Port=2
  VTQD_FrShaftSpd_rpm : Inport  Port=3
  VTQD_RrShaftSpd_rpm : Inport  Port=4
  AND1 : Logic  AllPortsSameDT=off  OutDataTypeStr=boolean
  AND3 : Logic  AllPortsSameDT=off  OutDataTypeStr=boolean
  Abs1 : Abs
  Abs2 : Abs
  Constant1 : Constant  Value=KTQD_PreLoadTqHold_rpm
  Constant16 : Constant  Value=KTQD_PreLoadTqHold_rpm
  Constant17 : Constant  Value=ZERO_FLOAT
  Constant2 : Constant  Value=ZERO_FLOAT
  MTQD_FrPreLoadTq_Y_Nm : Lookup_n-D  NumberOfTableDimensions=1  BreakpointsForDimension1=ATQD_FrPreLoadTq_X_s  Table=MTQD_FrPreLoadTq_Y_Nm  ExtrapMethod=Clip  InternalRulePriority=Speed  RndMeth=Simplest  InputSameDT=on
  MTQD_RrPreLoadTq_Y_Nm : Lookup_n-D  NumberOfTableDimensions=1  BreakpointsForDimension1=ATQD_FrPreLoadTq_X_s  Table=MTQD_RrPreLoadTq_Y_Nm  ExtrapMethod=Clip  InternalRulePriority=Speed  RndMeth=Simplest  InputSameDT=on
  NOT1 : Logic  Operator=NOT  AllPortsSameDT=off  OutDataTypeStr=boolean
  NOT6 : Logic  Operator=NOT  AllPortsSameDT=off  OutDataTypeStr=boolean
  Relational Operator1 : RelationalOperator  Operator=>  OutDataTypeStr=boolean  RndMeth=Simplest
  Relational Operator4 : RelationalOperator  Operator=>  OutDataTypeStr=boolean  RndMeth=Simplest
  SR_Latch1 : hcu_lib/Basic_Blocks/SR_Latch
  SR_Latch4 : hcu_lib/Basic_Blocks/SR_Latch
  Switch1 : Switch  Criteria=u2 ~= 0
  Switch6 : Switch  Criteria=u2 ~= 0
  VTQD_FrPreloadTq_Nm : Outport
  VTQD_RrPreloadTq_Nm : Outport  Port=2
  wires:
  [VTQD_RrPreloadTq_Nm] -> VTQD_RrPreloadTq_Nm/1
  [VTQD_FrPreloadTq_Nm] -> VTQD_FrPreloadTq_Nm/1
  VTQD_RrShaftSpd_rpm/1 -> [VTQD_RrShaftSpd_rpm]
  VTQD_FrShaftSpd_rpm/1 -> [VTQD_FrShaftSpd_rpm]
  VTQD_PreLoadHoldtime_s/1 -> [VTQD_PreLoadHoldtime_s]
  VTQD_PreLoadHold_flg/1 -> [VTQD_PreLoadHold_flg]
  SR_Latch1/1 -> Switch1/2
  [VTQD_RrShaftSpd_rpm] -> Abs1/1
  Switch1/1 -> [VTQD_RrPreloadTq_Nm]  "VTQD_RrPreloadTq_Nm"
  MTQD_RrPreLoadTq_Y_Nm/1 -> Switch1/3
  Constant2/1 -> Switch1/1
  [VTQD_PreLoadHoldtime_s] -> MTQD_RrPreLoadTq_Y_Nm/1
  NOT1/1 -> SR_Latch1/2
  Abs1/1 -> Relational Operator1/1
  Relational Operator1/1 -> AND1/2
  AND1/1 -> SR_Latch1/1
  Constant1/1 -> Relational Operator1/2
  [VTQD_PreLoadHold_flg] -> AND1/1
  [VTQD_PreLoadHold_flg] -> NOT1/1
  [VTQD_PreLoadHold_flg] -> AND3/1
  Constant16/1 -> Relational Operator4/2
  [VTQD_PreLoadHold_flg] -> NOT6/1
  SR_Latch4/1 -> Switch6/2
  MTQD_FrPreLoadTq_Y_Nm/1 -> Switch6/3
  [VTQD_PreLoadHoldtime_s] -> MTQD_FrPreLoadTq_Y_Nm/1
  NOT6/1 -> SR_Latch4/2
  AND3/1 -> SR_Latch4/1
  Relational Operator4/1 -> AND3/2
  Abs2/1 -> Relational Operator4/1
  Constant17/1 -> Switch6/1
  Switch6/1 -> [VTQD_FrPreloadTq_Nm]  "VTQD_FrPreloadTq_Nm"
  [VTQD_FrShaftSpd_rpm] -> Abs2/1

== system tqdtqr_rebuild_V3/Input_Convert/Main function/Front//Rear ramp parameters determine/Front First order filter input tau map and determination/Creep ==
  VTQR_FEDUWhlTqReqSmoothDelay_Nm : Inport
  VTQD_TqTargetShaftSpd_rpm : Inport  Port=2
  VVMC_EstSlope_Deg : Inport  Port=3
  Action Port : ActionPort  ActionPortLabel=elseif(u2 ~= 0)
  Data Type Conversion : DataTypeConversion  OutDataTypeStr=single
  Data Type Conversion1 : DataTypeConversion  OutDataTypeStr=single
  MTQR_CreepFEDUTs_Z_c : Lookup_n-D  BreakpointsForDimension1=ATQR_CreepFEDUTs_Y_Nm  BreakpointsForDimension2=ATQR_CreepFEDUTs_X_rpm  Table=MTQR_CreepFEDUTs_Z_c  ExtrapMethod=Clip  InternalRulePriority=Speed  RndMeth=Simplest  InputSameDT=on
      settings: InputPortMap=u0,u1
  MTQR_CreepGradeFEDUTs_Z_c : Lookup_n-D  BreakpointsForDimension1=ATQR_CreepGradeFEDUTs_Y_Deg  BreakpointsForDimension2=ATQR_CreepGradeFEDUTs_X_rpm  Table=MTQR_CreepGradeFEDUTs_Z_c  ExtrapMethod=Clip  InternalRulePriority=Speed  RndMeth=Simplest  InputSameDT=on
      settings: InputPortMap=u0,u1
  Min : MinMax  Inputs=2
  VTQR_CreepFEDUTs_c : Outport
  wires:
  MTQR_CreepFEDUTs_Z_c/1 -> [VTQR_CreepFEDUTs_c]  "VTQR_CreepFEDUTs_c"
  [VTQR_CreepFEDUTs_c] -> Data Type Conversion/1
  VTQR_FEDUWhlTqReqSmoothDelay_Nm/1 -> [VTQR_FEDUWhlTqReqSmoothDelay_Nm]
  VTQD_TqTargetShaftSpd_rpm/1 -> [VTQD_TqTargetShaftSpd_rpm]
  VVMC_EstSlope_Deg/1 -> [VVMC_EstSlope_Deg]
  [VTQD_TqTargetShaftSpd_rpm] -> MTQR_CreepFEDUTs_Z_c/2
  [VTQR_FEDUWhlTqReqSmoothDelay_Nm] -> MTQR_CreepFEDUTs_Z_c/1
  [VTQD_TqTargetShaftSpd_rpm] -> MTQR_CreepGradeFEDUTs_Z_c/2
  MTQR_CreepGradeFEDUTs_Z_c/1 -> [VTQR_CreepGradeFEDUTs_c]  "VTQR_CreepGradeFEDUTs_c"
  [VVMC_EstSlope_Deg] -> MTQR_CreepGradeFEDUTs_Z_c/1
  [VTQR_CreepGradeFEDUTs_c] -> Data Type Conversion1/1
  Min/1 -> VTQR_CreepFEDUTs_c/1
  Data Type Conversion/1 -> Min/1
  Data Type Conversion1/1 -> Min/2

== system tqdtqr_rebuild_V3/Input_Convert/Main function/Front//Rear ramp parameters determine/Front First order filter input tau map and determination/Drive mode ==
  VTQR_FEDUTs_c : Inport
  Action Port : ActionPort  ActionPortLabel=else
  VTQR_OutFEDUTs_c : Outport
  wires:
  VTQR_FEDUTs_c/1 -> VTQR_OutFEDUTs_c/1

== system tqdtqr_rebuild_V3/Input_Convert/Main function/Front//Rear ramp parameters determine/Front First order filter input tau map and determination/Preleoad ==
  KTQR_PreLoadTs_c : Inport
  Action Port : ActionPort  ActionPortLabel=elseif(u5~=0)
  VTQR_PreLoadTs_c : Outport
  wires:
  KTQR_PreLoadTs_c/1 -> VTQR_PreLoadTs_c/1

== system tqdtqr_rebuild_V3/Input_Convert/Main function/Front//Rear ramp parameters determine/Front First order filter input tau map and determination/PreleoadPreEn ==
  KTQR_PreLoadPreEnTs_c : Inport
  Action Port : ActionPort  ActionPortLabel=elseif(u6~=0)
  VTQR_PreLoadPreEnTs_c : Outport
  wires:
  KTQR_PreLoadPreEnTs_c/1 -> VTQR_PreLoadPreEnTs_c/1

== system tqdtqr_rebuild_V3/Input_Convert/Main function/Front//Rear ramp parameters determine/Front First order filter input tau map and determination/RDCActive ==
  VTQD_RegenMode_enum : Inport
  VVMC_ActMaxSlideRate_pct : Inport  Port=2
  Action Port : ActionPort  ActionPortLabel=if(u1~= 0)
  Data Type Conversion : DataTypeConversion  OutDataTypeStr=single
  Data Type Conversion1 : DataTypeConversion  OutDataTypeStr=single
  MTQR_AltRDCActiveFEDUTs_Z_c : Lookup_n-D  BreakpointsForDimension1=ATQR_AltRDCActiveFEDUTs_Y_enum  BreakpointsForDimension2=ATQR_AltRDCActiveFEDUTs_X_pct  Table=MTQR_AltRDCActiveFEDUTs_Z_c  TableDataTypeStr=Inherit: Inherit from 'Table data'  ExtrapMethod=Clip  InternalRulePriority=Speed  RndMeth=Simplest  InputSameDT=on
      settings: InputPortMap=u0,u1
  VTQR_RDCActiveFEDUTs_c : Outport
  wires:
  VVMC_ActMaxSlideRate_pct/1 -> MTQR_AltRDCActiveFEDUTs_Z_c/2
  VTQD_RegenMode_enum/1 -> Data Type Conversion/1
  Data Type Conversion/1 -> MTQR_AltRDCActiveFEDUTs_Z_c/1
  MTQR_AltRDCActiveFEDUTs_Z_c/1 -> [VTQR_RDCActiveFEDUTs_c]  "VTQR_RDCActiveFEDUTs_c"
  [VTQR_RDCActiveFEDUTs_c] -> Data Type Conversion1/1
  Data Type Conversion1/1 -> VTQR_RDCActiveFEDUTs_c/1

== system tqdtqr_rebuild_V3/Input_Convert/Main function/Front//Rear ramp parameters determine/Front First order filter input tau map and determination/TIP ==
  VTQD_TqTargetShaftSpd_rpm : Inport
  Action Port : ActionPort  ActionPortLabel=elseif(u4~=0)
  Data Type Conversion : DataTypeConversion  OutDataTypeStr=single
  MTQR_FEDUTIPOutTs_Y_c : Lookup_n-D  NumberOfTableDimensions=1  BreakpointsForDimension1=ATQR_FEDUTIPOutTs_X_rpm  Table=MTQR_FEDUTIPOutTs_Y_c  ExtrapMethod=Clip  InternalRulePriority=Speed  RndMeth=Simplest  InputSameDT=on
  VTQR_FEDUTIPOutTs_c : Outport
  wires:
  VTQD_TqTargetShaftSpd_rpm/1 -> MTQR_FEDUTIPOutTs_Y_c/1
  MTQR_FEDUTIPOutTs_Y_c/1 -> [VTQR_FEDUTIPOutTs_c]  "VTQR_FEDUTIPOutTs_c"
  [VTQR_FEDUTIPOutTs_c] -> Data Type Conversion/1
  Data Type Conversion/1 -> VTQR_FEDUTIPOutTs_c/1

== system tqdtqr_rebuild_V3/Input_Convert/Main function/Front//Rear ramp parameters determine/Front First order filter input tau map and determination/VMC ==
  VTQR_FEDUWhlTqReqSmoothDelay_Nm : Inport
  VTQD_TqTargetShaftSpd_rpm : Inport  Port=2
  Action Port : ActionPort  ActionPortLabel=elseif( u3 ~= 0)
  Data Type Conversion : DataTypeConversion  OutDataTypeStr=single
  MTQR_VMCFEDUTs_Z_c : Lookup_n-D  BreakpointsForDimension1=ATQR_VMCFEDUTs_Y_Nm  BreakpointsForDimension2=ATQR_VMCFEDUTs_X_rpm  Table=MTQR_VMCFEDUTs_Z_c  ExtrapMethod=Clip  InternalRulePriority=Speed  RndMeth=Simplest  InputSameDT=on
      settings: InputPortMap=u0,u1
  VTQR_VMCFEDUTs_c : Outport
  wires:
  VTQR_FEDUWhlTqReqSmoothDelay_Nm/1 -> MTQR_VMCFEDUTs_Z_c/1
  VTQD_TqTargetShaftSpd_rpm/1 -> MTQR_VMCFEDUTs_Z_c/2
  MTQR_VMCFEDUTs_Z_c/1 -> [VTQR_VMCFEDUTs_c]  "VTQR_VMCFEDUTs_c"
  [VTQR_VMCFEDUTs_c] -> Data Type Conversion/1
  Data Type Conversion/1 -> VTQR_VMCFEDUTs_c/1

== system tqdtqr_rebuild_V3/Input_Convert/Main function/Front//Rear ramp parameters determine/Front wheel rate limit determination/Drive mode ==
  VTQR_DriveModeTqIncDec_Nm : Inport
  Action Port : ActionPort  ActionPortLabel=else
  VTQR_OutDriveModeTqIncDec_Nm : Outport
  wires:
  VTQR_DriveModeTqIncDec_Nm/1 -> VTQR_OutDriveModeTqIncDec_Nm/1

== system tqdtqr_rebuild_V3/Input_Convert/Main function/Front//Rear ramp parameters determine/Front wheel rate limit determination/VTQD_OutFrZeroPointIncDec_Nm ==
  VTQD_FrZeroPointIncDec_Nm : Inport
  Action Port : ActionPort  ActionPortLabel=if(u1~= 0)
  VTQD_OutFrZeroPointIncDec_Nm : Outport
  wires:
  VTQD_FrZeroPointIncDec_Nm/1 -> VTQD_OutFrZeroPointIncDec_Nm/1

== system tqdtqr_rebuild_V3/Input_Convert/Main function/Front//Rear ramp parameters determine/Front wheel rate limit determination/VTQR_CreepFEDUTqIncDecSR_Nm ==
  VTQR_FEDUWhlTqReqSmoothDelay_Nm : Inport
  VTQD_TqTargetShaftSpd_rpm : Inport  Port=2
  VVMC_EstSlope_Deg : Inport  Port=3
  Action Port : ActionPort  ActionPortLabel=elseif(u2 ~= 0)
  Data Type Conversion : DataTypeConversion  OutDataTypeStr=single
  Data Type Conversion1 : DataTypeConversion  OutDataTypeStr=single
  MTQR_CreepFEDUTqDecSR_Z_Nm : Lookup_n-D  BreakpointsForDimension1=ATQR_CreepFEDUTqIncSR_Y_Nm  BreakpointsForDimension2=ATQR_CreepFEDUTqIncSR_X_rpm  Table=MTQR_CreepFEDUTqDecSR_Z_Nm  ExtrapMethod=Clip  InternalRulePriority=Speed  RndMeth=Simplest  InputSameDT=on
      settings: InputPortMap=u0,u1
  MTQR_CreepFEDUTqIncSR_Z_Nm : Lookup_n-D  BreakpointsForDimension1=ATQR_CreepFEDUTqIncSR_Y_Nm  BreakpointsForDimension2=ATQR_CreepFEDUTqIncSR_X_rpm  Table=MTQR_CreepFEDUTqIncSR_Z_Nm  ExtrapMethod=Clip  InternalRulePriority=Speed  RndMeth=Simplest  InputSameDT=on
      settings: InputPortMap=u0,u1
  MTQR_CreepGradeFTqDecSR_Z_c : Lookup_n-D  BreakpointsForDimension1=ATQR_CreepGradeRTqIncSR_Y_Deg  BreakpointsForDimension2=ATQR_CreepGradeRTqIncSR_X_rpm  Table=MTQR_CreepGradeFTqDecSR_Z_c  ExtrapMethod=Clip  InternalRulePriority=Speed  RndMeth=Simplest  InputSameDT=on
      settings: InputPortMap=u0,u1
  MTQR_CreepGradeFTqIncSR_Z_c : Lookup_n-D  BreakpointsForDimension1=ATQR_CreepGradeRTqIncSR_Y_Deg  BreakpointsForDimension2=ATQR_CreepGradeRTqIncSR_X_rpm  Table=MTQR_CreepGradeFTqIncSR_Z_c  ExtrapMethod=Clip  InternalRulePriority=Speed  RndMeth=Simplest  InputSameDT=on
      settings: InputPortMap=u0,u1
  Mux : Mux  Inputs=2
  Product : Product
  Product1 : Product
  VTQR_CreepFEDUTqIncDecSR_Nm : Outport
  wires:
  VTQR_FEDUWhlTqReqSmoothDelay_Nm/1 -> [VTQR_FEDUWhlTqReqSmoothDelay_Nm]
  VTQD_TqTargetShaftSpd_rpm/1 -> [VTQD_TqTargetShaftSpd_rpm]
  [VTQR_FEDUWhlTqReqSmoothDelay_Nm] -> MTQR_CreepFEDUTqIncSR_Z_Nm/1
  [VTQD_TqTargetShaftSpd_rpm] -> MTQR_CreepFEDUTqIncSR_Z_Nm/2
  [VTQR_FEDUWhlTqReqSmoothDelay_Nm] -> MTQR_CreepFEDUTqDecSR_Z_Nm/1
  [VTQD_TqTargetShaftSpd_rpm] -> MTQR_CreepFEDUTqDecSR_Z_Nm/2
  [VTQR_CreepFEDUTqIncSR_Nm] -> Data Type Conversion/1
  [VTQR_CreepFEDUTqDecSR_Nm] -> Data Type Conversion1/1
  Mux/1 -> VTQR_CreepFEDUTqIncDecSR_Nm/1
  Data Type Conversion1/1 -> Mux/2
  Data Type Conversion/1 -> Mux/1
  [VTQD_TqTargetShaftSpd_rpm] -> MTQR_CreepGradeFTqDecSR_Z_c/2
  MTQR_CreepGradeFTqDecSR_Z_c/1 -> [VTQR_CreepGradeFTqDecSR_c]  "VTQR_CreepGradeFTqDecSR_c"
  MTQR_CreepGradeFTqIncSR_Z_c/1 -> [VTQR_CreepGradeFTqIncSR_c]  "VTQR_CreepGradeFTqIncSR_c"
  [VTQD_TqTargetShaftSpd_rpm] -> MTQR_CreepGradeFTqIncSR_Z_c/2
  [VVMC_EstSlope_Deg] -> MTQR_CreepGradeFTqIncSR_Z_c/1
  [VVMC_EstSlope_Deg] -> MTQR_CreepGradeFTqDecSR_Z_c/1
  MTQR_CreepFEDUTqIncSR_Z_Nm/1 -> Product1/1
  Product1/1 -> [VTQR_CreepFEDUTqIncSR_Nm]  "VTQR_CreepFEDUTqIncSR_Nm"
  [VTQR_CreepGradeFTqIncSR_c] -> Product1/2
  MTQR_CreepFEDUTqDecSR_Z_Nm/1 -> Product/1
  Product/1 -> [VTQR_CreepFEDUTqDecSR_Nm]  "VTQR_CreepFEDUTqDecSR_Nm"
  [VTQR_CreepGradeFTqDecSR_c] -> Product/2
  VVMC_EstSlope_Deg/1 -> [VVMC_EstSlope_Deg]

== system tqdtqr_rebuild_V3/Input_Convert/Main function/Front//Rear ramp parameters determine/Front wheel rate limit determination/VTQR_FrPreLoadTqIncDec_Nm ==
  VTQR_FEDUWhlTqReqSmoothDelay_Nm : Inport
  VTQD_TqTargetShaftSpd_rpm : Inport  Port=2
  Action Port : ActionPort  ActionPortLabel=elseif( u3 ~= 0)
  Data Type Conversion1 : DataTypeConversion  OutDataTypeStr=single
  Data Type Conversion2 : DataTypeConversion  OutDataTypeStr=single
  MTQR_FrPreLoadTqDecSR_Z_Nm : Lookup_n-D  BreakpointsForDimension1=ATQR_FrPreLoadTqIncSR_Y_Nm  BreakpointsForDimension2=ATQR_FrPreLoadTqIncSR_X_rpm  Table=MTQR_FrPreLoadTqDecSR_Z_Nm  ExtrapMethod=Clip  InternalRulePriority=Speed  RndMeth=Simplest  InputSameDT=on
      settings: InputPortMap=u0,u1
  MTQR_FrPreLoadTqIncSR_Z_Nm : Lookup_n-D  BreakpointsForDimension1=ATQR_FrPreLoadTqIncSR_Y_Nm  BreakpointsForDimension2=ATQR_FrPreLoadTqIncSR_X_rpm  Table=MTQR_FrPreLoadTqIncSR_Z_Nm  ExtrapMethod=Clip  InternalRulePriority=Speed  RndMeth=Simplest  InputSameDT=on
      settings: InputPortMap=u0,u1
  Mux : Mux  Inputs=2
  VTQR_FrPreLoadTqIncDec_Nm : Outport
  wires:
  Mux/1 -> VTQR_FrPreLoadTqIncDec_Nm/1
  VTQD_TqTargetShaftSpd_rpm/1 -> [VTQD_TqTargetShaftSpd_rpm]
  VTQR_FEDUWhlTqReqSmoothDelay_Nm/1 -> [VTQR_FEDUWhlTqReqSmoothDelay_Nm]
  MTQR_FrPreLoadTqIncSR_Z_Nm/1 -> [VTQR_FrPreLoadTqIncSR_Nm]  "VTQR_FrPreLoadTqIncSR_Nm"
  MTQR_FrPreLoadTqDecSR_Z_Nm/1 -> [VTQR_FrPreLoadTqDecSR_Nm]  "VTQR_FrPreLoadTqDecSR_Nm"
  [VTQR_FEDUWhlTqReqSmoothDelay_Nm] -> MTQR_FrPreLoadTqIncSR_Z_Nm/1
  [VTQD_TqTargetShaftSpd_rpm] -> MTQR_FrPreLoadTqIncSR_Z_Nm/2
  [VTQR_FEDUWhlTqReqSmoothDelay_Nm] -> MTQR_FrPreLoadTqDecSR_Z_Nm/1
  [VTQD_TqTargetShaftSpd_rpm] -> MTQR_FrPreLoadTqDecSR_Z_Nm/2
  [VTQR_FrPreLoadTqIncSR_Nm] -> Data Type Conversion1/1
  Data Type Conversion1/1 -> Mux/1
  [VTQR_FrPreLoadTqDecSR_Nm] -> Data Type Conversion2/1
  Data Type Conversion2/1 -> Mux/2
